simulink model "H8_6GDL"  (R2022b)
settings: Solver=VariableStepAuto  StartTime=0.0  StopTime=10.0  RelTol=1e-3
InitFcn:
  | m = 200;
  | g = 9.81;
  | 
  | x_lev12 = 0.443;
  | x_lev34 = 0.542;
  | x_guid12 = 0.4475;
  | x_guid34 = 0.5465;
  | x_lim = 0.0495;
  | 
  | y_lev13 = 0.23686;
  | y_lev24 = 0.23686;
  | y_guid13 = 0.24263;
  | y_guid24 = 0.24263;
  | y_lim = 0.0005;
  | y_brk = 0.21552;
  | 
  | z_lev = 0.08546;
  | z_guid = 0.026;
  | z_lim = 0.1055;
  | z_brk = 0.03941;
  | 
  | kp_lev = 50;
  | ki_lev = 400;
  | kp_guid = 50;
  | ki_guid = 400;
  | 
  | Imax_lev = 50;
  | Imin_lev = -50;
  | Imax_guid = 50;
  | Imin_guid = 0;
  | 
  | cg_nom = 0.567;
  | 
  | I = [43.082 0 0; 0 26.887 -0; 0 0 29.297]
values from neighbouring files (symbols this model uses):
  Ka = [34.5916764023 4.46928641015 34.7816336405 4.65924364837 92.2484067139 -92.2484067139 74.2332308826 -74.2332308826 -4220.94514487 -4209.6309051 -4205.06787146 -4193.7536317 ... (120 elements, 8x15)]    [Ka.mat]    (also in linealizacion_5gdl_bien.m = place(Aa,Ba,[ -1.5 -1.5 -1.5 -1.5 -2 -2 -6 -6 -7 -7 -5 -5 -2; linealizacion_EMS.m = place(Aa,Ba,[ -1 -1 -2 -2 -3 -3 -6 -6 -7 -7 -5 -5 -4 -4 -5 -)
settings Model: Creator=USUARIO  LastModifiedBy=aceao

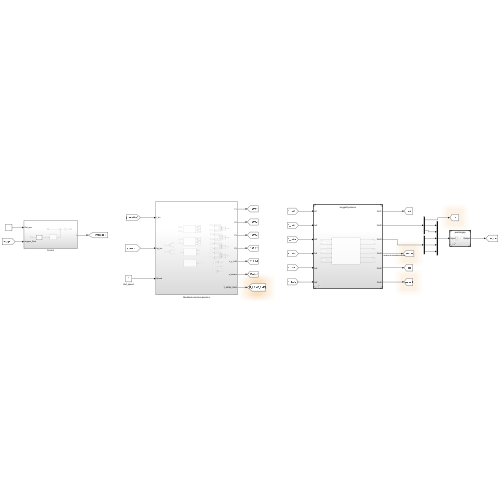
[thumbnail: Simulink's stored preview of the top-level diagram]
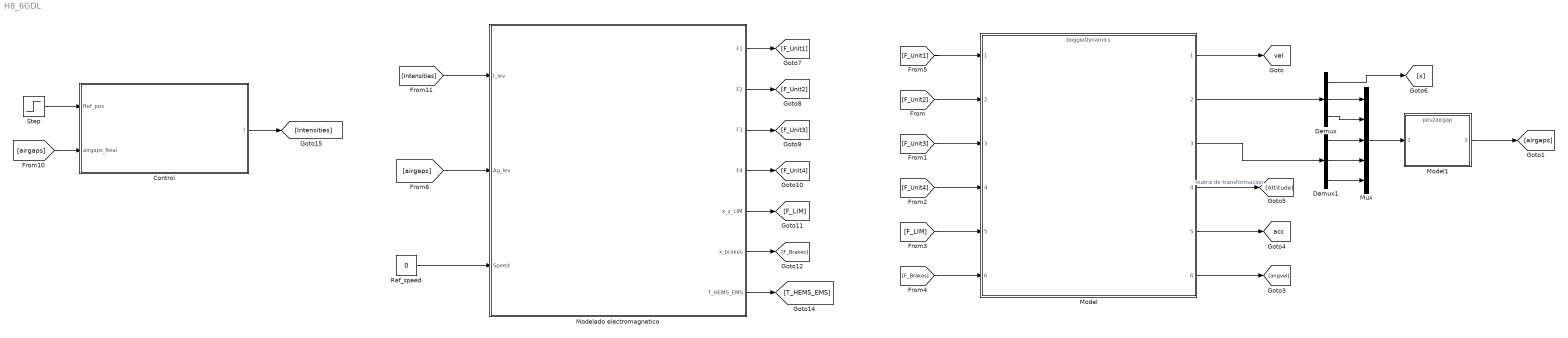
== system H8_6GDL ==
  Control : Subsystem
  Demux : Demux  Outputs=3
  Demux1 : Demux  Outputs=3
  Model : ModelReference  ModelNameDialog=boggieDynamics.mdl  SimulationMode=Normal  ModelReferenceVersion=1.17
  Model1 : ModelReference  ModelNameDialog=pos2airgap.slx  SimulationMode=Normal  ModelReferenceVersion=1.2
  Modelado electromagnetico : Subsystem
  Mux : Mux  Inputs=5
  Ref_speed : Constant  Value=0
  Step : Step  SampleTime=0
  tag scope: acc=global, vel=global
  wires:
  [F_Unit4] -> Model/4
  [F_Unit3] -> Model/3
  [F_LIM] -> Model/5
  [F_Unit2] -> Model/2
  [F_Brakes] -> Model/6
  Model/4 -> [Attitude]  "matriz de transformacion"
  [F_Unit1] -> Model/1
  Model/3 -> Demux1/1
  Mux/1 -> Model1/1
  Model/2 -> Demux/1
  Demux/3 -> Mux/2
  Demux/1 -> [x]
  Model/1 -> [vel]
  Demux/2 -> Mux/1
  Model/5 -> [acc]
  Model/6 -> [angvel]
  Ref_speed/1 -> Modelado electromagnetico/3(Speed)
  [airgaps] -> Modelado electromagnetico/2(Ag_lev)
  [Intensities] -> Modelado electromagnetico/1(I_lev)
  Modelado electromagnetico/6(x_brakes) -> [F_Brakes]
  Modelado electromagnetico/5(x_y_LIM) -> [F_LIM]
  Modelado electromagnetico/4(F4) -> [F_Unit4]
  Modelado electromagnetico/3(F3) -> [F_Unit3]
  Modelado electromagnetico/2(F2) -> [F_Unit2]
  Modelado electromagnetico/1(F1) -> [F_Unit1]
  Modelado electromagnetico/7(T_HEMS_EMS) -> [T_HEMS_EMS]
  [airgaps] -> Control/2(airgaps_Real)
  Control/1(I) -> [Intensities]
  Step/1 -> Control/1(Ref_pos)
  Demux1/1 -> Mux/3
  Demux1/2 -> Mux/4
  Demux1/3 -> Mux/5
  Model1/1 -> [airgaps]

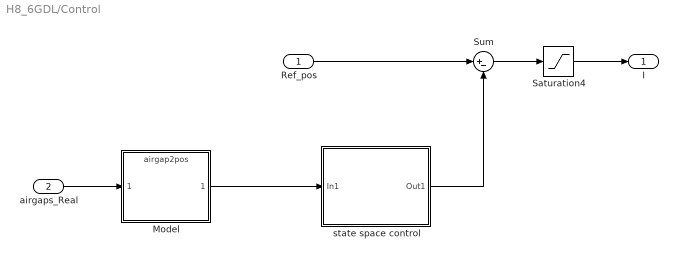
== system H8_6GDL/Control ==
  Ref_pos : Inport
  airgaps_Real : Inport  Port=2
  Model : ModelReference  ModelNameDialog=airgap2pos.slx  SimulationMode=Normal  ModelReferenceVersion=1.2
  Saturation4 : Saturate  UpperLimit=55  LowerLimit=-55
  Sum : Sum  Inputs=|+-
  state space control : Subsystem
  I : Outport
  wires:
  airgaps_Real/1 -> Model/1
  Ref_pos/1 -> Sum/1
  Sum/1 -> Saturation4/1
  Saturation4/1 -> I/1
  Model/1 -> state space control/1(In1)
  state space control/1(Out1) -> Sum/2

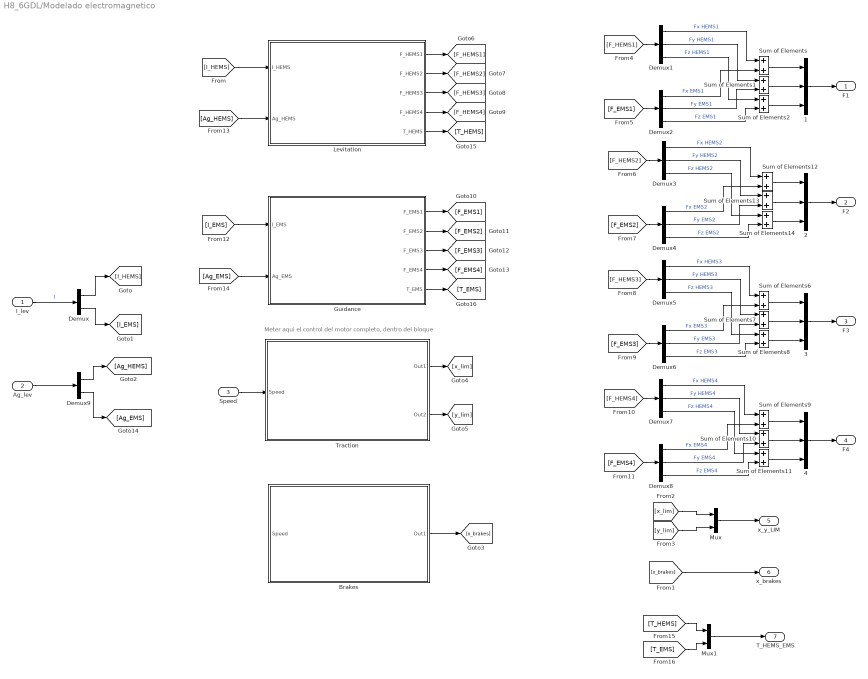
== system H8_6GDL/Modelado electromagnetico ==
  note: Meter aqui el control del motor completo, dentro del bloque
  I_lev : Inport
  Ag_lev : Inport  Port=2
  Speed : Inport  Port=3
  {1..4} (4 alike) : Mux  Inputs=3
  Brakes : Subsystem
  Demux : Demux  Outputs=2
  Demux{1..8} (8 alike) : Demux  Outputs=3
  Demux9 : Demux  Outputs=2
  Guidance : Subsystem
  Levitation : Subsystem
  Mux : Mux  Inputs=2
  Mux1 : Mux  Inputs=2
  Sum of Elements{,1..2,6..14} (12 alike) : Sum
  Traction : Subsystem
  F1 : Outport
  F2 : Outport  Port=2
  F3 : Outport  Port=3
  F4 : Outport  Port=4
  x_y_LIM : Outport  Port=5
  x_brakes : Outport  Port=6
  T_HEMS_EMS : Outport  Port=7
  wires:
  I_lev/1 -> Demux/1  "I"
  Demux/1 -> [I_HEMS]
  Demux/2 -> [I_EMS]
  [I_HEMS] -> Levitation/1(I_HEMS)
  Brakes/1(Out1) -> [x_brakes]
  [x_brakes] -> x_brakes/1
  Traction/1(Out1) -> [x_lim]
  Traction/2(Out2) -> [y_lim]
  Mux/1 -> x_y_LIM/1
  [x_lim] -> Mux/1
  [y_lim] -> Mux/2
  Levitation/1(F_HEMS1) -> [F_HEMS1]
  Levitation/2(F_HEMS2) -> [F_HEMS2]
  Levitation/3(F_HEMS3) -> [F_HEMS3]
  Levitation/4(F_HEMS4) -> [F_HEMS4]
  Sum of Elements/1 -> 1/1
  1/1 -> F1/1
  Sum of Elements1/1 -> 1/2
  Sum of Elements2/1 -> 1/3
  2/1 -> F2/1
  [F_HEMS1] -> Demux1/1
  Demux1/1 -> Sum of Elements/1  "Fx HEMS1"
  Demux1/2 -> Sum of Elements1/1  "Fy HEMS1"
  Demux1/3 -> Sum of Elements2/1  "Fz HEMS1"
  3/1 -> F3/1
  Sum of Elements8/1 -> 3/3
  Sum of Elements6/1 -> 3/1
  Sum of Elements7/1 -> 3/2
  4/1 -> F4/1
  Sum of Elements11/1 -> 4/3
  Sum of Elements9/1 -> 4/1
  Sum of Elements10/1 -> 4/2
  Guidance/2(F_EMS2) -> [F_EMS2]
  Guidance/3(F_EMS3) -> [F_EMS3]
  Guidance/4(F_EMS4) -> [F_EMS4]
  Guidance/1(F_EMS1) -> [F_EMS1]
  Demux2/1 -> Sum of Elements/2  "Fx EMS1"
  [F_EMS1] -> Demux2/1
  Demux2/2 -> Sum of Elements1/2  "Fy EMS1"
  Demux2/3 -> Sum of Elements2/2  "Fz EMS1"
  [F_EMS2] -> Demux4/1
  Demux4/1 -> Sum of Elements12/2  "Fx EMS2"
  Demux4/2 -> Sum of Elements13/2  "Fy EMS2"
  Sum of Elements14/1 -> 2/3
  Demux3/1 -> Sum of Elements12/1  "Fx HEMS2"
  [F_HEMS2] -> Demux3/1
  Demux3/2 -> Sum of Elements13/1  "Fy HEMS2"
  Demux3/3 -> Sum of Elements14/1  "Fz HEMS2"
  Sum of Elements13/1 -> 2/2
  Sum of Elements12/1 -> 2/1
  Demux4/3 -> Sum of Elements14/2  "Fz EMS2"
  Demux5/3 -> Sum of Elements8/1  "Fz HEMS3"
  Demux5/2 -> Sum of Elements7/1  "Fy HEMS3"
  [F_HEMS3] -> Demux5/1
  Demux6/3 -> Sum of Elements8/2  "Fz EMS3"
  [F_EMS3] -> Demux6/1
  Demux6/1 -> Sum of Elements6/2  "Fx EMS3"
  Demux5/1 -> Sum of Elements6/1  "Fx HEMS3"
  Demux6/2 -> Sum of Elements7/2  "Fy EMS3"
  Demux7/3 -> Sum of Elements11/1  "Fz HEMS4"
  Demux8/3 -> Sum of Elements11/2  "Fz EMS4"
  Demux8/2 -> Sum of Elements10/2  "Fy EMS4"
  Demux7/2 -> Sum of Elements10/1  "Fy HEMS4"
  Demux7/1 -> Sum of Elements9/1  "Fx HEMS4"
  Demux8/1 -> Sum of Elements9/2  "Fx EMS4"
  [F_HEMS4] -> Demux7/1
  [F_EMS4] -> Demux8/1
  [I_EMS] -> Guidance/1(I_EMS)
  Ag_lev/1 -> Demux9/1
  Demux9/1 -> [Ag_HEMS]
  Demux9/2 -> [Ag_EMS]
  [Ag_HEMS] -> Levitation/2(Ag_HEMS)
  [Ag_EMS] -> Guidance/2(Ag_EMS)
  Levitation/5(T_HEMS) -> [T_HEMS]
  Speed/1 -> Traction/1(Speed)
  Guidance/5(T_EMS) -> [T_EMS]
  Mux1/1 -> T_HEMS_EMS/1
  [T_HEMS] -> Mux1/1
  [T_EMS] -> Mux1/2

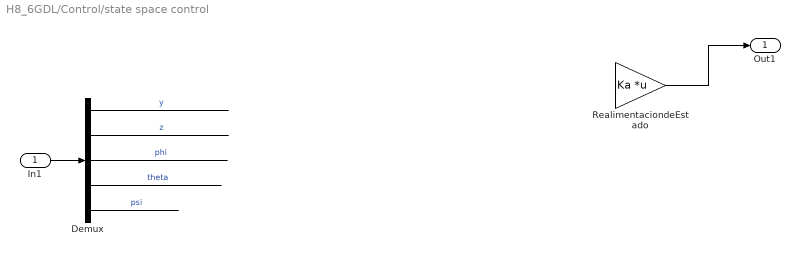
== system H8_6GDL/Control/state space control ==
  In1 : Inport
  Demux : Demux  Outputs=5
  RealimentaciondeEstado : Gain  Gain=Ka  Multiplication=Matrix(K*u)
  Out1 : Outport
  wires:
  In1/1 -> Demux/1
  RealimentaciondeEstado/1 -> Out1/1
  Demux/1 -> ?  "y"
  Demux/2 -> ?  "z"
  Demux/3 -> ?  "phi"
  Demux/4 -> ?  "theta"
  Demux/5 -> ?  "psi"

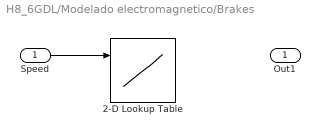
== system H8_6GDL/Modelado electromagnetico/Brakes ==
  Speed : Inport
  2-D Lookup Table : Lookup_n-D  BreakpointsForDimension1=[1:3]  BreakpointsForDimension2=[1:3]  InternalRulePriority=Speed  RndMeth=Simplest
      settings: InputPortMap=u0,u1
  Out1 : Outport
  wires:
  Speed/1 -> 2-D Lookup Table/1

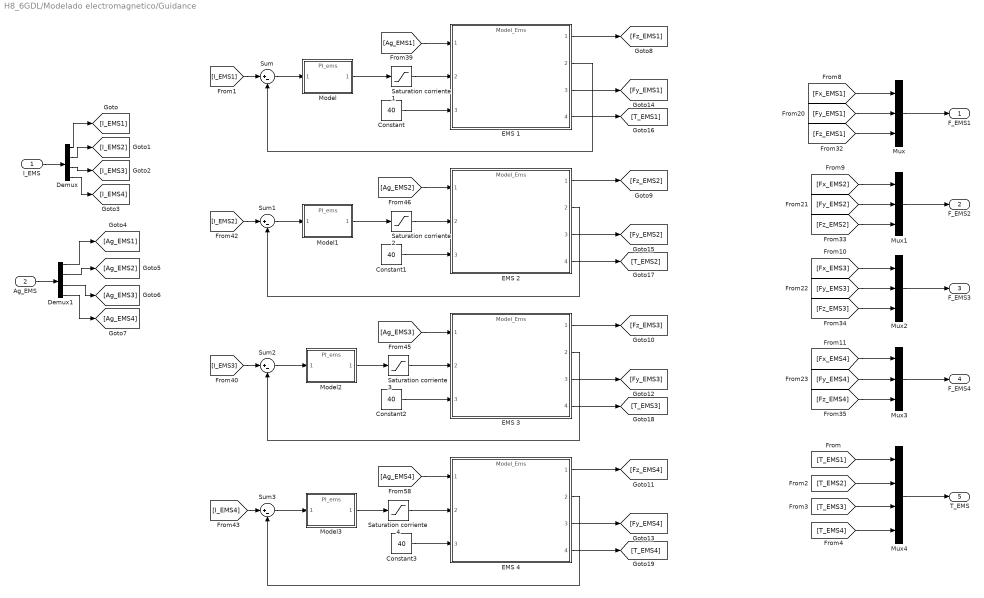
== system H8_6GDL/Modelado electromagnetico/Guidance ==
  I_EMS : Inport
  Ag_EMS : Inport  Port=2
  Constant{,1..3} (4 alike) : Constant  Value=40
  Demux : Demux
  Demux1 : Demux
  EMS {1..4} (4 alike) : ModelReference  ModelNameDialog=Model_Ems.slx  SimulationMode=Normal  ModelReferenceVersion=1.20
  Model{,1..3} (4 alike) : ModelReference  ModelNameDialog=PI_ems.slx  SimulationMode=Normal  ModelReferenceVersion=1.1
  Mux{,1..3} (4 alike) : Mux  Inputs=3
  Mux4 : Mux
  Saturation corriente {1..4} (4 alike) : Saturate  UpperLimit=Imax_guid  LowerLimit=Imin_guid
  Sum{,1..3} (4 alike) : Sum  Inputs=|+-
  F_EMS1 : Outport
  F_EMS2 : Outport  Port=2
  F_EMS3 : Outport  Port=3
  F_EMS4 : Outport  Port=4
  T_EMS : Outport  Port=5
  wires:
  [Fz_EMS4] -> Mux3/3
  Demux1/4 -> [Ag_EMS4]
  [Fy_EMS1] -> Mux/2
  I_EMS/1 -> Demux/1
  Mux1/1 -> F_EMS2/1
  Demux/2 -> [I_EMS2]
  [Fy_EMS3] -> Mux2/2
  Mux3/1 -> F_EMS4/1
  [Fy_EMS4] -> Mux3/2
  [Fz_EMS1] -> Mux/3
  Mux/1 -> F_EMS1/1
  Mux2/1 -> F_EMS3/1
  [Fx_EMS3] -> Mux2/1
  Demux1/3 -> [Ag_EMS3]
  Ag_EMS/1 -> Demux1/1
  [Fz_EMS3] -> Mux2/3
  Demux/1 -> [I_EMS1]
  [Fz_EMS2] -> Mux1/3
  [Fx_EMS1] -> Mux/1
  Demux1/1 -> [Ag_EMS1]
  Demux/4 -> [I_EMS4]
  [Fx_EMS2] -> Mux1/1
  [Fy_EMS2] -> Mux1/2
  [Fx_EMS4] -> Mux3/1
  Demux/3 -> [I_EMS3]
  Demux1/2 -> [Ag_EMS2]
  EMS 1/3 -> [Fy_EMS1]
  [Ag_EMS4] -> EMS 4/1
  EMS 4/3 -> [Fy_EMS4]
  EMS 4/1 -> [Fz_EMS4]
  EMS 2/1 -> [Fz_EMS2]
  EMS 1/2 -> Sum/2
  EMS 3/1 -> [Fz_EMS3]
  [Ag_EMS3] -> EMS 3/1
  Constant1/1 -> EMS 2/3
  Constant3/1 -> EMS 4/3
  Constant2/1 -> EMS 3/3
  Constant/1 -> EMS 1/3
  EMS 1/1 -> [Fz_EMS1]
  [Ag_EMS2] -> EMS 2/1
  Model/1 -> Saturation corriente 1/1
  EMS 3/3 -> [Fy_EMS3]
  EMS 2/3 -> [Fy_EMS2]
  [Ag_EMS1] -> EMS 1/1
  Sum/1 -> Model/1
  Sum1/1 -> Model1/1
  EMS 2/2 -> Sum1/2
  [I_EMS2] -> Sum1/1
  Model1/1 -> Saturation corriente 2/1
  [I_EMS1] -> Sum/1
  Sum2/1 -> Model2/1
  EMS 3/2 -> Sum2/2
  [I_EMS3] -> Sum2/1
  Model2/1 -> Saturation corriente 3/1
  Sum3/1 -> Model3/1
  EMS 4/2 -> Sum3/2
  [I_EMS4] -> Sum3/1
  Model3/1 -> Saturation corriente 4/1
  Mux4/1 -> T_EMS/1
  EMS 1/4 -> [T_EMS1]
  EMS 2/4 -> [T_EMS2]
  EMS 3/4 -> [T_EMS3]
  EMS 4/4 -> [T_EMS4]
  [T_EMS1] -> Mux4/1
  [T_EMS2] -> Mux4/2
  [T_EMS3] -> Mux4/3
  [T_EMS4] -> Mux4/4
  Saturation corriente 1/1 -> EMS 1/2
  Saturation corriente 2/1 -> EMS 2/2
  Saturation corriente 3/1 -> EMS 3/2
  Saturation corriente 4/1 -> EMS 4/2

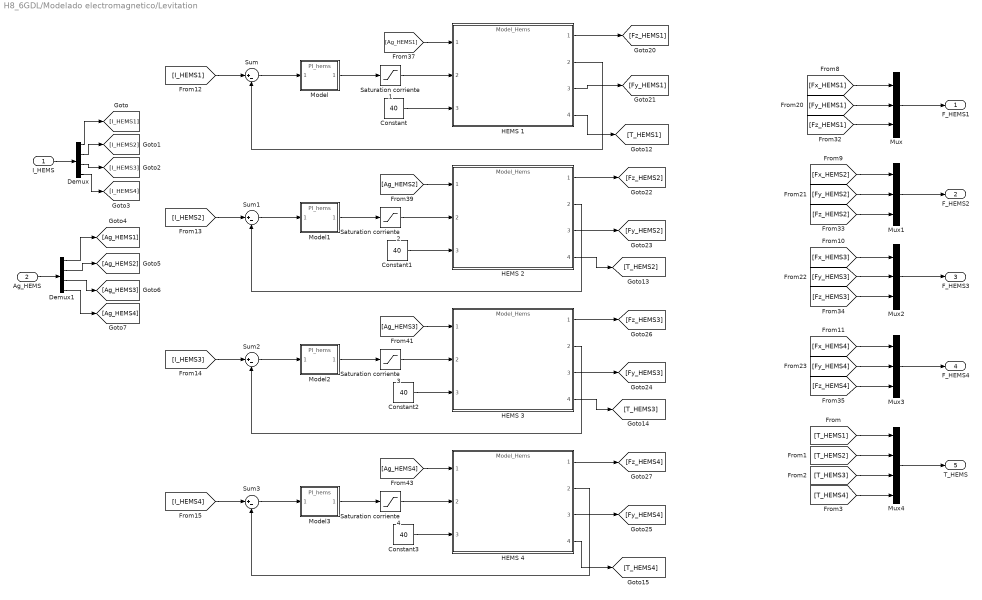
== system H8_6GDL/Modelado electromagnetico/Levitation ==
  I_HEMS : Inport
  Ag_HEMS : Inport  Port=2
  Constant{,1..3} (4 alike) : Constant  Value=40
  Demux : Demux
  Demux1 : Demux
  HEMS {1..4} (4 alike) : ModelReference  ModelNameDialog=Model_Hems.slx  SimulationMode=Normal  ModelReferenceVersion=1.15
  Model{,1..3} (4 alike) : ModelReference  ModelNameDialog=PI_hems.slx  SimulationMode=Normal  ModelReferenceVersion=1.1
  Mux{,1..3} (4 alike) : Mux  Inputs=3
  Mux4 : Mux
  Saturation corriente {1..4} (4 alike) : Saturate  UpperLimit=Imax_lev  LowerLimit=Imin_lev
  Sum{,1..3} (4 alike) : Sum  Inputs=|+-
  F_HEMS1 : Outport
  F_HEMS2 : Outport  Port=2
  F_HEMS3 : Outport  Port=3
  F_HEMS4 : Outport  Port=4
  T_HEMS : Outport  Port=5
  wires:
  I_HEMS/1 -> Demux/1
  Mux/1 -> F_HEMS1/1
  Mux1/1 -> F_HEMS2/1
  Mux2/1 -> F_HEMS3/1
  Mux3/1 -> F_HEMS4/1
  Demux/1 -> [I_HEMS1]
  Demux/2 -> [I_HEMS2]
  Demux/3 -> [I_HEMS3]
  Demux/4 -> [I_HEMS4]
  Demux1/2 -> [Ag_HEMS2]
  Demux1/3 -> [Ag_HEMS3]
  Ag_HEMS/1 -> Demux1/1
  Demux1/4 -> [Ag_HEMS4]
  Demux1/1 -> [Ag_HEMS1]
  [Fx_HEMS1] -> Mux/1
  [Fx_HEMS2] -> Mux1/1
  [Fx_HEMS3] -> Mux2/1
  [Fx_HEMS4] -> Mux3/1
  [Fy_HEMS1] -> Mux/2
  [Fy_HEMS2] -> Mux1/2
  [Fy_HEMS3] -> Mux2/2
  [Fy_HEMS4] -> Mux3/2
  [Fz_HEMS1] -> Mux/3
  [Fz_HEMS2] -> Mux1/3
  [Fz_HEMS3] -> Mux2/3
  [Fz_HEMS4] -> Mux3/3
  Model/1 -> Saturation corriente 1/1
  [Ag_HEMS1] -> HEMS 1/1
  HEMS 1/1 -> [Fz_HEMS1]
  HEMS 1/3 -> [Fy_HEMS1]
  HEMS 2/3 -> [Fy_HEMS2]
  HEMS 2/1 -> [Fz_HEMS2]
  [Ag_HEMS2] -> HEMS 2/1
  Model1/1 -> Saturation corriente 2/1
  HEMS 3/3 -> [Fy_HEMS3]
  HEMS 3/1 -> [Fz_HEMS3]
  [Ag_HEMS3] -> HEMS 3/1
  Model2/1 -> Saturation corriente 3/1
  HEMS 4/3 -> [Fy_HEMS4]
  HEMS 4/1 -> [Fz_HEMS4]
  [Ag_HEMS4] -> HEMS 4/1
  Model3/1 -> Saturation corriente 4/1
  Constant1/1 -> HEMS 2/3
  Constant2/1 -> HEMS 3/3
  Constant3/1 -> HEMS 4/3
  HEMS 1/2 -> Sum/2
  Sum/1 -> Model/1
  Sum1/1 -> Model1/1
  HEMS 2/2 -> Sum1/2
  Sum2/1 -> Model2/1
  HEMS 3/2 -> Sum2/2
  Sum3/1 -> Model3/1
  HEMS 4/2 -> Sum3/2
  [I_HEMS1] -> Sum/1
  [I_HEMS2] -> Sum1/1
  [I_HEMS3] -> Sum2/1
  [I_HEMS4] -> Sum3/1
  HEMS 1/4 -> [T_HEMS1]
  Constant/1 -> HEMS 1/3
  HEMS 2/4 -> [T_HEMS2]
  HEMS 3/4 -> [T_HEMS3]
  HEMS 4/4 -> [T_HEMS4]
  Mux4/1 -> T_HEMS/1
  [T_HEMS1] -> Mux4/1
  [T_HEMS4] -> Mux4/4
  [T_HEMS3] -> Mux4/3
  [T_HEMS2] -> Mux4/2
  Saturation corriente 1/1 -> HEMS 1/2
  Saturation corriente 2/1 -> HEMS 2/2
  Saturation corriente 3/1 -> HEMS 3/2
  Saturation corriente 4/1 -> HEMS 4/2

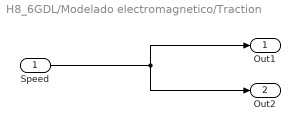
== system H8_6GDL/Modelado electromagnetico/Traction ==
  Speed : Inport
  Out1 : Outport
  Out2 : Outport  Port=2
  wires:
  Speed/1 -> Out1/1, Out2/1
